simulink model "speedL298_II"  (R2013b)
settings: Solver=FixedStepDiscrete  SolverMode=SingleTasking  StartTime=0.0  StopTime=inf  RelTol=1e-3
libraries: arduinolib x12, simulink x3
settings Model: SimulationMode=external  ExtModeTrigDuration=2  Creator=Joshua  LastModifiedBy=Joshua
settings OptimizationCC: OptimizeModelRefInitCode=on  LifeSpan=1
settings DebuggingCC: SolverPrmCheckMsg=none
settings HardwareCC: ProdBitPerInt=16  ProdBitPerPointer=8  ProdIntDivRoundTo=Zero  ProdEndianess=LittleEndian  ProdWordSize=8  ProdHWDeviceType=Atmel->AVR
settings RTWCC: SystemTargetFile=realtime.tlc  GenerateMakefile=off  TemplateMakefile=realtime.tmf  Description=Run on Target Hardware  RTWVerbose=off  ProcessScript=realtime_make_rtw_hook
settings STFCustomTargetCC: TargetLibSuffix=.a  GenerateSampleERTMain=on  ERTCustomFileBanners=on  SupportNonInlinedSFcns=off  SupportVariableSizeSignals=on  MATLABClassNameForMDSCustomization=Simulink.SoftwareTarget.ERTCustomization  GRTInterface=off  SystemTargetFile=realtime.tlc
settings ERTTargetCC: CodeReplacementLibrary=ANSI_C  GenerateSampleERTMain=on  ParMdlRefBuildCompliant=off  CompOptLevelCompliant=off  ConcurrentExecutionCompliant=off  CombineOutputUpdateFcns=off  ERTFirstTimeCompliant=off  SupportContinuousTime=on  SupportVariableSizeSignals=on  ModelStepFunctionPrototypeControlCompliant=off  CPPClassGenCompliant=off  ExtModeTransport=3  ExtModeMexFile=ext_serial_win32_comm  ExtModeMexArgs=0 1 9600  InlinedParameterPlacement=NonHierarchical  ERTSrcFileBannerTemplate=realtime_code_template.cgt  ERTHdrFileBannerTemplate=realtime_code_template.cgt  ERTDataSrcFileTemplate=realtime_code_template.cgt  ERTDataHdrFileTemplate=realtime_code_template.cgt  ERTCustomFileTemplate=realtime_file_process.tlc

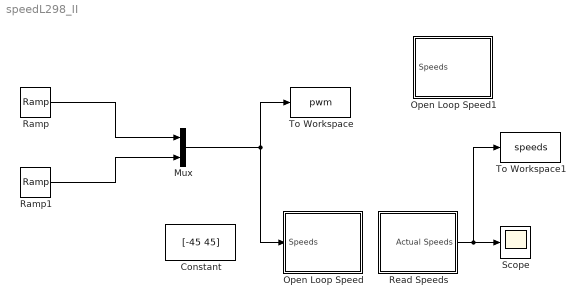
== system speedL298_II ==
  Constant : Constant  Value=[-45 45]
  Mux : Mux  Inputs=2
  Open Loop Speed : Subsystem
  Open Loop Speed1 : Subsystem
  Ramp : simulink/Sources/Ramp  slope=25.5  start=0  X0=0
  Ramp1 : simulink/Sources/Ramp  slope=-25.5  start=0  X0=0
  Read Speeds : Subsystem
  Scope : Scope
  To Workspace : ToWorkspace  VariableName=pwm  SampleTime=-1  SaveFormat=Timeseries
  To Workspace1 : ToWorkspace  VariableName=speeds  SampleTime=-1  SaveFormat=Timeseries
  wires:
  Read Speeds/1(Actual Speeds) -> To Workspace1/1, Scope/1
  Ramp/1 -> Mux/1
  Ramp1/1 -> Mux/2
  Mux/1 -> Open Loop Speed/1(Speeds), To Workspace/1

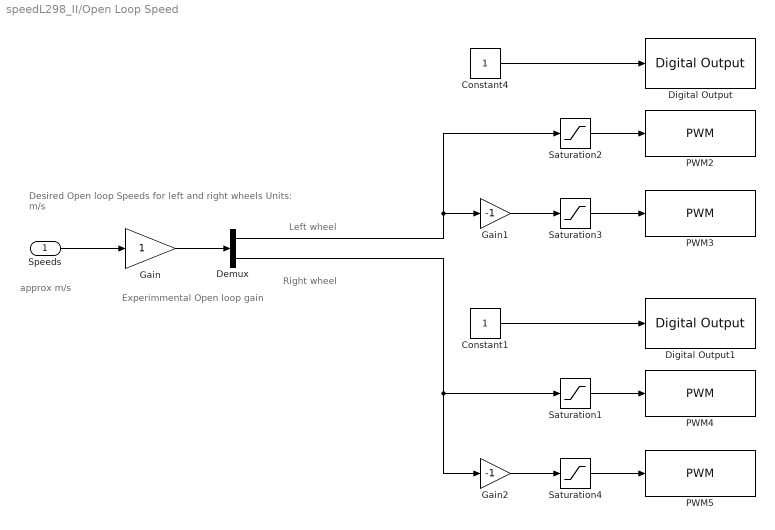
== system speedL298_II/Open Loop Speed ==
  note: Right wheel
  note: Left wheel
  note: approx m/s
  note: Experimmental
      | Open loop gain
  note: Desired Open loop Speeds for left and right wheels
      | Units: m/s
  Speeds : Inport
  Constant1 : Constant
  Constant4 : Constant
  Demux : Demux  Outputs=2
  Digital Output : arduinolib/Digital Output  pinNumber=8
  Digital Output1 : arduinolib/Digital Output  pinNumber=13
  Gain : Gain
  Gain1 : Gain  Gain=-1
  Gain2 : Gain  Gain=-1
  PWM2 : arduinolib/PWM  pinNumber=9
  PWM3 : arduinolib/PWM  pinNumber=10
  PWM4 : arduinolib/PWM  pinNumber=11
  PWM5 : arduinolib/PWM  pinNumber=12
  Saturation{1..4} (4 alike) : Saturate  UpperLimit=255  LowerLimit=0  OutDataTypeStr=uint8
  wires:
  Speeds/1 -> Gain/1
  Gain/1 -> Demux/1
  Constant1/1 -> Digital Output1/1
  Demux/1 -> Saturation2/1, Gain1/1
  Constant4/1 -> Digital Output/1
  Saturation2/1 -> PWM2/1
  Saturation3/1 -> PWM3/1
  Gain1/1 -> Saturation3/1
  Demux/2 -> Gain2/1, Saturation1/1
  Gain2/1 -> Saturation4/1
  Saturation1/1 -> PWM4/1
  Saturation4/1 -> PWM5/1

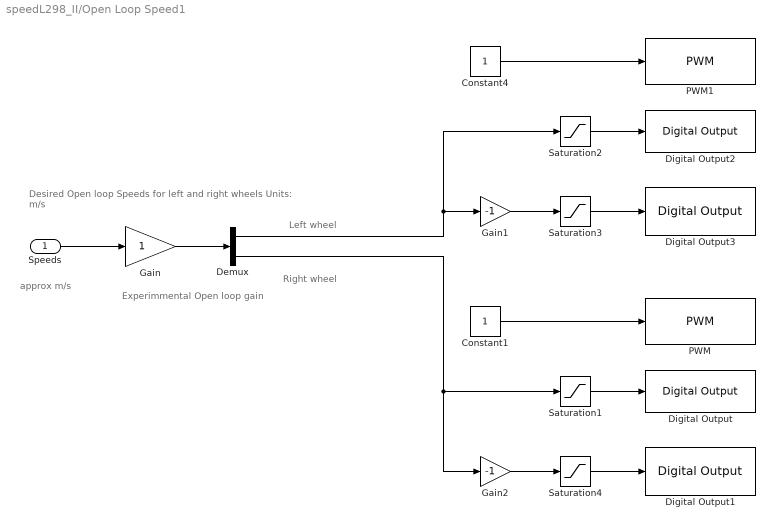
== system speedL298_II/Open Loop Speed1 ==
  note: Right wheel
  note: Left wheel
  note: approx m/s
  note: Experimmental
      | Open loop gain
  note: Desired Open loop Speeds for left and right wheels
      | Units: m/s
  Speeds : Inport
  Constant1 : Constant
  Constant4 : Constant
  Demux : Demux  Outputs=2
  Digital Output : arduinolib/Digital Output  pinNumber=11
  Digital Output1 : arduinolib/Digital Output  pinNumber=12
  Digital Output2 : arduinolib/Digital Output  pinNumber=9
  Digital Output3 : arduinolib/Digital Output  pinNumber=10
  Gain : Gain
  Gain1 : Gain  Gain=-1
  Gain2 : Gain  Gain=-1
  PWM : arduinolib/PWM  pinNumber=13
  PWM1 : arduinolib/PWM  pinNumber=8
  Saturation{1..4} (4 alike) : Saturate  UpperLimit=255  LowerLimit=0  OutDataTypeStr=uint8
  wires:
  Speeds/1 -> Gain/1
  Gain/1 -> Demux/1
  Constant1/1 -> PWM/1
  Demux/1 -> Saturation2/1, Gain1/1
  Constant4/1 -> PWM1/1
  Saturation2/1 -> Digital Output2/1
  Saturation3/1 -> Digital Output3/1
  Gain1/1 -> Saturation3/1
  Demux/2 -> Gain2/1, Saturation1/1
  Gain2/1 -> Saturation4/1
  Saturation1/1 -> Digital Output/1
  Saturation4/1 -> Digital Output1/1

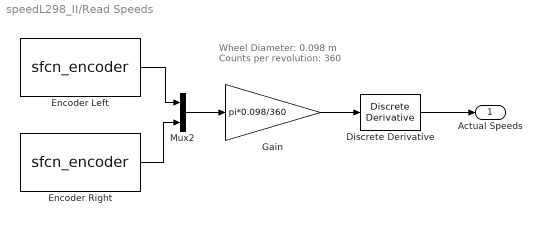
== system speedL298_II/Read Speeds ==
  note: Wheel Diameter: 0.098 m
      | Counts per revolution: 360
  Discrete Derivative : simulink/Discrete/Discrete Derivative  gainval=1.0  ICPrevScaledInput=0.0  InputProcessing=Inherited  OutMin=[]  OutMax=[]  OutDataType=fixdt(1, 16)  OutScaling=2^-10  DoSatur=off
  Encoder Left : S-Function  InitFcn=try, set_param(gcb,'FunctionName','sfcn_encoder'), end  FunctionName=sfcn_encoder  Parameters=uint8(0),uint8(3),uint8(2)  SFunctionModules=sfcn_encoder_wrapper  EnableBusSupport=off  mask(S-Function Builder){}
      mask init:
      | val = [[.9  0.75 0.75 1 1 .9 .9 1]',[1 1 0.75 0.75 .9 .9 1 .9]'];try , sys = get_param(gcb,'SfunBuilderFcnName');if isempty(sys), sys = get_param(gcb,'FunctionName'); end,catch, sys = get_param(gcb,'FunctionName'); end
      settings: CopyFcn=set_param(gcbh,'LinkStatus','none')  PreSaveFcn=try, set_param(gcb,'FunctionName','sfcn_encoder'), end  OpenFcn=sfunctionwizard(gcbh)
      mask Display: plot(val(:,1),val(:,2)),disp(sys), port_label('output',1,'pos')
  Encoder Right : S-Function  InitFcn=try, set_param(gcb,'FunctionName','sfcn_encoder'), end  FunctionName=sfcn_encoder  Parameters=uint8(1),uint8(19),uint8(18)  SFunctionModules=sfcn_encoder_wrapper  EnableBusSupport=off  mask(S-Function Builder){}
      mask init: same as speedL298_II/Read Speeds/Encoder Left
      settings: CopyFcn=set_param(gcbh,'LinkStatus','none')  PreSaveFcn=try, set_param(gcb,'FunctionName','sfcn_encoder'), end  OpenFcn=sfunctionwizard(gcbh)
      mask Display: plot(val(:,1),val(:,2)),disp(sys), port_label('output',1,'pos')
  Gain : Gain  Gain=pi*0.098/360  OutDataTypeStr=double
  Mux2 : Mux  Inputs=2
  Actual Speeds : Outport
  wires:
  Gain/1 -> Discrete Derivative/1
  Encoder Left/1 -> Mux2/1
  Encoder Right/1 -> Mux2/2
  Discrete Derivative/1 -> Actual Speeds/1
  Mux2/1 -> Gain/1
